simulink model "SOC_simulink"  (R2018a)
settings: Solver=FixedStepDiscrete  StartTime=0.0  StopTime=18000.0  FixedStep=1  RelTol=1e-3
undefined symbols (not defined in the file): DiscIntNeverNeededParam
settings Model: Creator=redou  LastModifiedBy=TRANSHOST

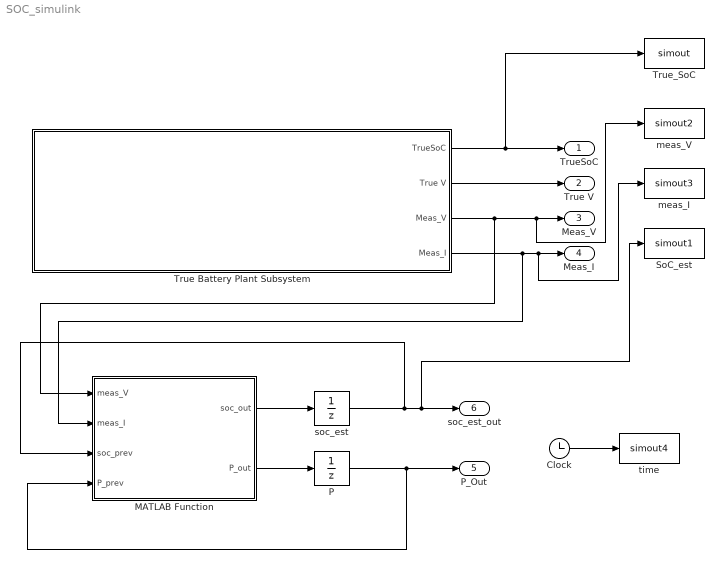
== system SOC_simulink ==
  Clock : Clock
  MATLAB Function : MATLAB Function  TreatAsAtomicUnit=on
  P : UnitDelay  InitialCondition=0.001  SampleTime=-1
  SoC_est : ToWorkspace  VariableName=simout1  SampleTime=-1
      settings: Save2DSignal=2-D array (concatenate along first dimension)
  True Battery Plant Subsystem : Subsystem
  True_SoC : ToWorkspace  VariableName=simout  SampleTime=-1
      settings: Save2DSignal=2-D array (concatenate along first dimension)
  meas_I : ToWorkspace  VariableName=simout3  SampleTime=-1
      settings: Save2DSignal=2-D array (concatenate along first dimension)
  meas_V : ToWorkspace  VariableName=simout2  SampleTime=-1
      settings: Save2DSignal=2-D array (concatenate along first dimension)
  soc_est : UnitDelay  InitialCondition=1  SampleTime=-1
  time : ToWorkspace  VariableName=simout4  SampleTime=-1
      settings: Save2DSignal=2-D array (concatenate along first dimension)
  TrueSoC : Outport
  True V : Outport  Port=2
  Meas_V : Outport  Port=3
  Meas_I : Outport  Port=4
  P_Out : Outport  Port=5
  "soc_est_out " : Outport  Port=6
  wires:
  True Battery Plant Subsystem/1(TrueSoC) -> True_SoC/1, TrueSoC/1
  True Battery Plant Subsystem/2(True V) -> True V/1
  True Battery Plant Subsystem/3(Meas_V) -> MATLAB Function/1(meas_V), Meas_V/1, meas_V/1
  True Battery Plant Subsystem/4(Meas_I) -> Meas_I/1, meas_I/1, MATLAB Function/2(meas_I)
  soc_est/1 -> MATLAB Function/3(soc_prev), SoC_est/1, "soc_est_out "/1
  P/1 -> MATLAB Function/4(P_prev), P_Out/1
  MATLAB Function/2(P_out) -> P/1
  MATLAB Function/1(soc_out) -> soc_est/1
  Clock/1 -> time/1

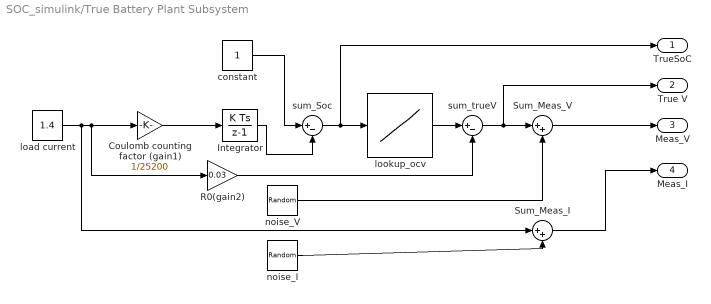
== system SOC_simulink/True Battery Plant Subsystem ==
  "                            Sum_Meas_I" : Sum  Inputs=|++
  "                           Sum_Meas_V" : Sum  Inputs=|++
  "                      sum_trueV" : Sum  Inputs=|+-
  "                  sum_Soc" : Sum  Inputs=|+-
  Coulomb counting factor (gain1) : Gain  Gain=1/25200
  Integrator : DiscreteIntegrator  SampleTime=-1  ICPrevOutput=DiscIntNeverNeededParam  ICPrevScaledInput=DiscIntNeverNeededParam
  R0(gain2) : Gain  Gain=0.03
  constant : Constant
  load current : Constant  Value=1.4
  lookup_ocv : Lookup_n-D  NumberOfTableDimensions=1  BreakpointsForDimension1=[-5:5]  Table=tanh([-5:5])  InternalRulePriority=Speed  RndMeth=Simplest  InputSameDT=on
  noise_I : RandomNumber  Variance=0.0001  SampleTime=1
  noise_V : RandomNumber  Variance=0.0004  SampleTime=1
  TrueSoC : Outport
  True V : Outport  Port=2
  Meas_V : Outport  Port=3
  Meas_I : Outport  Port=4
  wires:
  noise_V/1 -> "                           Sum_Meas_V"/2
  Coulomb counting factor (gain1)/1 -> Integrator/1
  constant/1 -> "                  sum_Soc"/1
  load current/1 -> "                            Sum_Meas_I"/1, Coulomb counting factor (gain1)/1, R0(gain2)/1
  "                  sum_Soc"/1 -> TrueSoC/1, lookup_ocv/1
  "                            Sum_Meas_I"/1 -> Meas_I/1
  "                      sum_trueV"/1 -> True V/1, "                           Sum_Meas_V"/1
  noise_I/1 -> "                            Sum_Meas_I"/2
  Integrator/1 -> "                  sum_Soc"/2
  R0(gain2)/1 -> "                      sum_trueV"/2
  lookup_ocv/1 -> "                      sum_trueV"/1
  "                           Sum_Meas_V"/1 -> Meas_V/1

== matlab function SOC_simulink/MATLAB Function ==
  data: meas_V input; soc_out output; meas_I input; soc_prev input; P_prev input; P_out output

function [soc_out, P_out] = skf_update(meas_V, meas_I, soc_prev, P_prev)
% Standard (Linear) Kalman Filter for a 12V 7Ah lead-acid battery.
% Estimates SoC from noisy voltage and current measurements using a
% linear approximation of the OCV-SoC characteristic.
%
% Inputs:
%   meas_V   - measured terminal voltage (V)
%   meas_I   - measured current (A), positive for discharge
%   soc_prev - previous SoC estimate (0 to 1)
%   P_prev   - previous error covariance
% Outputs:
%   soc_out  - updated SoC estimate (0 to 1)
%   P_out    - updated error covariance

% --- Battery parameters --------------------------------------------------
Q   = 7 * 3600;       % nominal capacity (As) -> 25200 As
R0  = 0.03;           % series resistance (Ohm)
dt  = 1;              % sample time (s)

% --- Linear OCV model: OCV = a * SoC + b --------------------------------
% Derived from experimental OCV data (SoC range 0.2-0.9)
a = 1.0789;           % slope (V per unit SoC)
b = 11.6462;          % intercept (V)

% --- Filter tuning -------------------------------------------------------
Q_proc = 1e-12;       % process noise covariance (SoC variance)
R_meas = 0.0004;      % measurement noise variance (sigma_V^2 = 0.02^2)
P_min  = 1e-8;        % covariance lower bound

% --- Prediction (Coulomb counting) ---------------------------------------
soc_pred = soc_prev - (meas_I * dt) / Q;
P_pred   = P_prev + Q_proc;

% --- Measurement update --------------------------------------------------
% Predicted terminal voltage using the linear OCV model
V_pred = a * soc_pred + b - meas_I * R0;

% Measurement sensitivity (constant)
H = a;

% Innovation (voltage residual)
innov = meas_V - V_pred;

% Kalman gain (scalar because the state is scalar SoC)
S = H * P_pred * H + R_meas;
K = P_pred * H / S;

% Corrected state and covariance
soc_out = soc_pred + K * innov;
P_out   = (1 - K * H) * P_pred;

% Clamp covariance to avoid numerical issues
if P_out < P_min
    P_out = P_min;
end
end
